simulink model "tb_SYSTEM"  (R2022b)
settings: Solver=FixedStepDiscrete  StartTime=0  StopTime=0.01  RelTol=1e-3
InitFcn:
  | init_SYSTEM;
values from neighbouring files (symbols this model uses):
  AD9545_INIT = bitconcat(ufi(AD9545_tmp(:,1),16,0),ufi(AD9545_tmp(:,2),8,0))    [init_SYSTEM.m]
  AXI_DDR_CONTROL = Simulink.Parameter    [init_SYSTEM.m]
  AXI_MonADC_CONTROL = Simulink.Parameter    [init_SYSTEM.m]
  AXI_MonADC_SPI_Wr = Simulink.Parameter    [init_SYSTEM.m]
  AXI_PWR_CONTROL = Simulink.Parameter    [init_SYSTEM.m]
  AXI_XAVIER_CONTROL = Simulink.Parameter    [init_SYSTEM.m]
  model_time_step = 1/80e6    (= 1.25e-08)    [init_CameraIO.m]    (also in init_SYSTEM.m)
libraries: hdlsllib x22, simulink x20
(part 2 of 2)

== stateflow chart tb_SYSTEM/SYSTEM/AD9545CC/init ==
  settings: executeAtInitialization=1
  state UPD_REG
    en:
    push = true;
    data_out = ufi(0x000F01,24,0);
    ex:
    push = false;
  note: 60 ms min reset;
      | 125 ticks per us
  state INIT
    en:
    init_cnt = 0;
    push = false;
    du:
    if fifo_empty
    push = true;
    init_cnt = init_cnt + 1;
    data_out = data_init(init_cnt);
    else
    push = false;
    end
    ex:
    push = false;
  state WAIT0
  state RESET
    data_out = ufi(0,24,0);
    init_cnt = uint16(0);
    init_sz = uint16(length(data_init));
    push = false;
    data_in_prev = ufi(0,24,0);
    resetn = false;
    init_done = false;
  state WAIT3
    resetn = true;
  state CAL
    en:
    init_cnt = 0;
    du:
    push = true;
    switch init_cnt
    case 0
    data_out = ufi(0x200000,24,0);
    case 1
    data_out = ufi(0x000F01,24,0);
    case 2
    data_out = ufi(0x200002,24,0);
    case 3
    data_out = ufi(0x000F01,24,0);
    end
    init_cnt = init_cnt + 1;
    ex:
    push = false;
  state WAIT01
  state INF
    en:
    data_in_prev = data_in;
    push = false;
    du:
    if data_in_prev ~= data_in
    push = true;
    else
    push = false;
    end
    data_in_prev = data_in;
    data_out = data_in;
    ex:
    push = false;
  state WAIT1
  state INIT_DONE
    init_done = true;
  (default) -> RESET
  WAIT0 -> UPD_REG : [fifo_empty]
  INIT -> WAIT0 : [init_cnt == init_sz]
  UPD_REG -> WAIT01
  WAIT3 -> INIT : after(10000*125,tick)
  RESET -> WAIT3 : after(70000*125,tick)
  INF -> INIT : [rst]
  WAIT01 -> CAL : [fifo_empty]
  CAL -> WAIT1 : [init_cnt == 4]
  INIT_DONE -> INF
  WAIT1 -> INIT_DONE : [fifo_empty]
  data: data_init input fixdt(0,24,0); push output boolean; init_cnt local uint16; data_out output fixdt(0,24,0); data_in input fixdt(0,24,0); data_in_prev local fixdt(0,24,0); resetn output boolean; init_sz local uint16; fifo_empty input boolean; init_done output boolean; rst input boolean

== stateflow chart tb_SYSTEM/SYSTEM/AD9545CC/spi_sm ==
  settings: executeAtInitialization=1
  state RESET
    nCS = ufi(1,1,0);
    SCK = ufi(1,1,0);
    MOSI = ufi(0,1,0);
    cnt_clk = uint8(0);
    cnt_bit = uint8(0);
    dout = ufi(0,24,0);
    din = ufi(0,24,0);
    data_out = ufi(0,24,0);
  state ONE_BIT
    cnt_clk = cnt_clk - 1;
    din = din;
    if bitget(din,cnt_bit) == 1
    MOSI = 1;
    else
    MOSI = 0;
    end
    if cnt_clk > bitshift(clk_len,-1)
    SCK = 0;
    else
    SCK = 1;
    end
    dout = bitset(dout, cnt_bit, MISO);
  state IDLE
    nCS = 1;
    SCK = 1;
    MOSI = 0;
    cnt_clk = clk_len;
    cnt_bit = bit_len;
    din = data_in;
    data_out = dout;
  state WAIT
    en:
    stop = true;
    du:
    stop = false;
  (default) -> RESET
  ONE_BIT -> (junction 7) : [cnt_clk == 0]
      | {cnt_clk = clk_len; cnt_bit = cnt_bit - 1;}
  IDLE -> ONE_BIT : [start]
      | {nCS = 0; dout = 0; din = data_in;}
  RESET -> IDLE
  (junction 7) -> ONE_BIT [order 2]
  (junction 7) -> WAIT [order 1] : [cnt_bit == 0]
      | {nCS = 1; data_out = dout; stop = true;}
  WAIT -> IDLE : after(clk_len,tick)
  data: data_in input fixdt(0,24,0); nCS output fixdt(0,1,0); MOSI output fixdt(0,1,0); cnt_clk local uint8; cnt_bit local uint8; MISO input fixdt(0,1,0); din local fixdt(0,24,0); data_out output fixdt(0,24,0); dout local fixdt(0,24,0); SCK output fixdt(0,1,0); bit_len constant uint8 =24; clk_len constant uint8 =8; start input boolean; stop output boolean

== stateflow chart tb_SYSTEM/SYSTEM/spi2axil/AXI4LiteMaster ==
  settings: executeAtInitialization=1
  state RESET
    rd_avalid = false;
    wr_valid = false;
    rd_addr = uint32(0);
    rd_len = uint8(1);
    wr_addr = uint32(0);
    wr_len = uint8(1);
    wr_data = uint32(0);
  state IDLE
  state WR_READY
  state WR_VALID
    en:
    wr_valid = true;
    ex:
    wr_valid = false;
  state RD_AVALID
    rd_avalid = true;
  state RD_AREADY
  state RD_DVALID
    rd_avalid = false;
  (default) -> RESET
  IDLE -> WR_READY [order 1] : [wvalid]
      | {wr_addr = waddr;
      | wr_data = wdata;}
  WR_READY -> WR_VALID : [wr_ready]
  WR_VALID -> IDLE
  RESET -> IDLE
  RD_AREADY -> RD_AVALID : [rd_aready]
  IDLE -> RD_AREADY [order 2] : [rvalid]
      | {rd_addr = raddr;}
  RD_AVALID -> RD_DVALID
  RD_DVALID -> IDLE : [rd_dvalid]
  data: rd_aready input boolean; rd_addr output uint32; rd_len output uint8; rd_avalid output boolean; rd_dvalid input boolean; wr_addr output uint32; wr_valid output boolean; wr_len output uint8; wr_data output uint32; wr_ready input boolean; wvalid input boolean; wdata input uint32; waddr input uint32; rvalid input boolean; raddr input uint32

== stateflow chart tb_SYSTEM/SYSTEM/SPISlave/spi_slave ==
  settings: executeAtInitialization=1
  state READY
    if cbit == nbit
    if cword == 0
    if bitand(drecvd,uint32(0x3)) == 0
    waddr = bitand(drecvd,0xFFFFFFFC);
    next_data_write = true;
    else
    rvalid = true;
    raddr = bitand(drecvd,0xFFFFFFFC);
    next_data_write = false;
    end
    elseif next_data_write
    wvalid = true;
    wdata = drecvd;
    if cword > 1
    waddr = waddr + 4;
    end
    end
    end
    cword = cword + 1;
    cbit = 0;
  state RESET
    MISO = false;
    cbit = uint8(0);
    cword = uint8(0);
    drecvd = uint32(0);
    next_data_write = false;
    wvalid = false;
    waddr = uint32(0);
    wdata = uint32(0);
    rvalid = false;
    raddr = uint32(0);
  state IDLE
    cbit = 0;
    wvalid = false;
    rvalid = false;
    next_data_write = false;
    cword = 0;
    MISO = false;
  state CLK_HIGH_WAIT
    if cbit < nbit
    drecvd = bitset(drecvd, cbit+1, MOSI);
    if bitget(rdata,cbit+1) == 1
    MISO = true;
    else
    MISO = false;
    end
    end
  state CLK_LOW_WAIT
    ex:
    cbit = cbit + 1;
  CLK_LOW_WAIT -> READY [order 2] : [nCS]
  READY -> IDLE [order 1] : [nCS]
  READY -> CLK_HIGH_WAIT [order 2] : [~nCS]
      | {wvalid = false;
      | rvalid = false;}
  CLK_HIGH_WAIT -> READY [order 1] : [nCS | cbit == nbit]
  (default) -> RESET
  CLK_HIGH_WAIT -> CLK_LOW_WAIT [order 2] : [SCK]
  RESET -> IDLE
  IDLE -> CLK_HIGH_WAIT : [~nCS]
  CLK_LOW_WAIT -> CLK_HIGH_WAIT [order 1] : [~SCK]
  data: nCS input boolean; MOSI input boolean; MISO output boolean; SCK input boolean; cbit local uint8; wvalid output boolean; rvalid output boolean; wdata output uint32; waddr output uint32; raddr output uint32; drecvd local uint32; rdata input uint32; nbit constant uint8 =32; next_data_write local boolean; cword local uint8
